simulink model "Full_stack_ADMM"  (R2022b)
settings: Solver=VariableStepAuto  StartTime=0.0  StopTime=inf  RelTol=1e-3
libraries: modbusMatLib x12
settings Model: Creator=pppc  LastModifiedBy=pppc
settings SolverCC: AlgebraicLoopSolver=TrustRegion
settings DebuggingCC: UnconnectedInputMsg=warning  UnconnectedOutputMsg=warning  UnconnectedLineMsg=warning  SFMachineParentedDataDiag=warning
settings ModelReferenceCC: EnableRefExpFcnMdlSchedulingChecks=on
settings RTWCC: DLArmComputeVersion=19.05

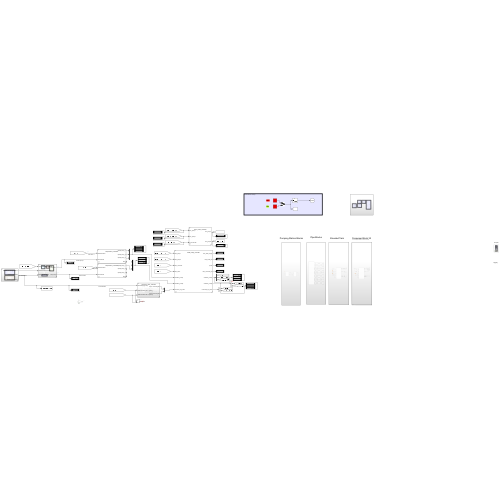
[thumbnail: Simulink's stored preview of the top-level diagram]
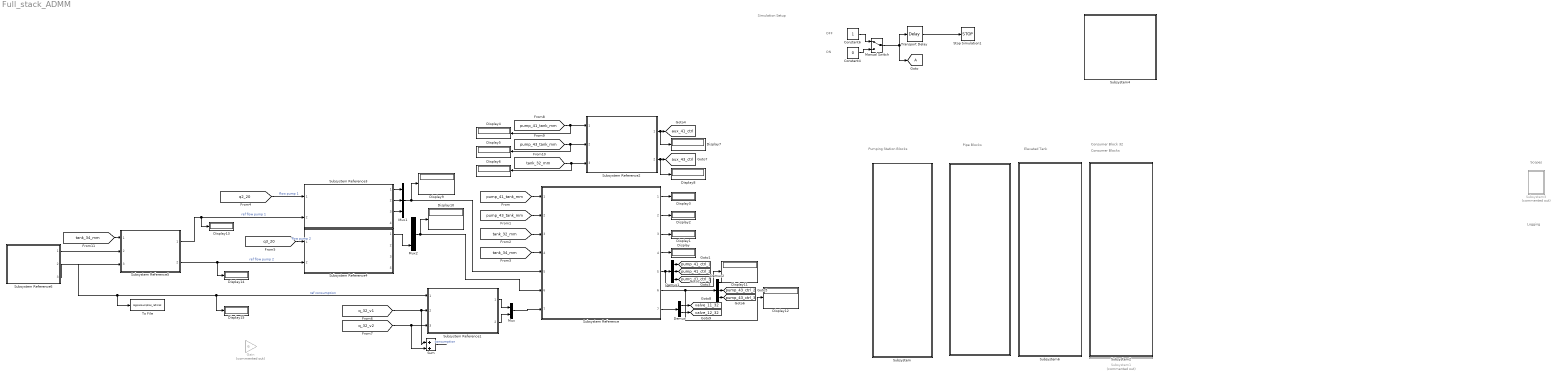
== system Full_stack_ADMM ==
  note: Logging
  note: Scopes
  note: Pumping Station Blocks
  note: OFF
  note: ON
  note: Simulation Setup
  note: Consumer Blocks
  note: Pipe Blocks
  note: Elevated Tank
  note: Consumer Block 32
  " " : Subsystem
  Constant4 : Constant  Value=0
  Constant6 : Constant
  Demux : Demux  Outputs=2
  Demux1 : Demux  Outputs=3
  Demux2 : Demux  Outputs=3
  Display{,1..15} (16 alike) : Display
  Gain : Gain  Commented=on  Gain=6
  Goto : Goto  TagVisibility=global
  Manual Switch : ManualSwitch
  Mux : Mux  Inputs=2
  Mux1 : Mux  Inputs=3
  Mux2 : Mux  Inputs=3
  Stop Simulation1 : Stop
  Subsystem : Subsystem
  Subsystem Reference : Subsystem  ReferencedSubsystem=WDN_safety_controller  consumer_tank_max=575  consumer_tank_min=75  pump_tank_min=125
  Subsystem Reference1 : Subsystem  ReferencedSubsystem=consumer_valve_controller
  Subsystem Reference2 : Subsystem  ReferencedSubsystem=reutrn_water_controller  tank_pump_max=530  consumer_min=75  consumer_max=570  switch_time=60  tank_pump_ref=400
  Subsystem Reference3 : Subsystem  ReferencedSubsystem=Pumpstation_Controller  Speedlimit_Upper=95  Speedlimit_Lower=65  TotalPumps=3  Kp=6.5  Ki=3.25
  Subsystem Reference4 : Subsystem  ReferencedSubsystem=Pumpstation_Controller  Speedlimit_Upper=95  Speedlimit_Lower=65  TotalPumps=1  Kp=16  Ki=2
  Subsystem Reference5 : Subsystem  ReferencedSubsystem=consensusADMM
  Subsystem Reference6 : Subsystem  ReferencedSubsystem=DemandEletricityPrice
  Subsystem1 : Subsystem  Commented=on
  Subsystem2 : Subsystem
  Subsystem3 : Subsystem  Commented=on
  Subsystem4 : Subsystem
  Subsystem6 : Subsystem
  Sum : Sum  Inputs=|++
  To File : ToFile  Filename=log\consumption_ref.mat  MatrixName=con_ref  SaveFormat=Timeseries
  Transport Delay : TransportDelay  DelayTime=2
  tag scope: aux_41_ctrl=global, aux_43_ctrl=global, pump_41_ctrl_1=global, pump_41_ctrl_2=global, pump_41_ctrl_3=global, pump_43_ctrl_2=global, pump_43_ctrl_3=global, valve_11_32=global, valve_12_32=global
  wires:
  Constant4/1 -> Manual Switch/2
  Transport Delay/1 -> Stop Simulation1/1
  Constant6/1 -> Manual Switch/1
  Manual Switch/1 -> Goto/1, Transport Delay/1
  Subsystem Reference1/1 -> Mux/1
  Subsystem Reference1/2 -> Mux/2
  Mux/1 -> Subsystem Reference/7
  Subsystem Reference/7 -> Demux/1
  Subsystem Reference3/2 -> Mux1/2
  Subsystem Reference3/1 -> Mux1/1
  Subsystem Reference3/3 -> Mux1/3
  Mux2/1 -> Display10/1, Subsystem Reference/6
  Mux1/1 -> Subsystem Reference/5, Display9/1
  Subsystem Reference5/2 -> Display14/1, Subsystem Reference4/2  "ref flow pump 2"
  Subsystem Reference5/1 -> Display13/1, Subsystem Reference3/2  "ref flow pump 1"
  Subsystem Reference6/1 -> Subsystem Reference5/2
  Subsystem Reference6/3 -> Subsystem Reference5/3
  [pump_41_tank_mm] -> Subsystem Reference/1
  [pump_43_tank_mm] -> Subsystem Reference/2
  [tank_32_mm] -> Subsystem Reference/3
  [tank_34_mm] -> Subsystem Reference/4
  [q2_20] -> Subsystem Reference3/1  "flow pump 1"
  [q3_20] -> Subsystem Reference4/1  "flow pump 2"
  [q_32_v1] -> Sum/1, Subsystem Reference1/2
  [q_32_v2] -> Sum/2, Subsystem Reference1/3
  [pump_41_tank_mm] -> Display4/1, Subsystem Reference2/1
  [pump_43_tank_mm] -> Display5/1, Subsystem Reference2/2
  [tank_32_mm] -> Display6/1, Subsystem Reference2/3
  Subsystem Reference/5 -> Display11/1, Demux1/1
  Demux1/1 -> [pump_41_ctrl_1]
  Demux1/2 -> [pump_41_ctrl_2]
  Demux1/3 -> [pump_41_ctrl_3]
  [tank_34_mm] -> Subsystem Reference5/1
  Demux2/3 -> [pump_43_ctrl_3]
  Subsystem Reference/6 -> Demux2/1, Display12/1
  Demux2/1 -> ?
  Demux2/2 -> [pump_43_ctrl_2]
  Subsystem Reference/4 -> Display/1
  Subsystem Reference/3 -> Display1/1
  Subsystem Reference/2 -> Display2/1
  Subsystem Reference/1 -> Display3/1
  Subsystem Reference2/1 -> Display7/1, [aux_41_ctrl]
  Subsystem Reference2/2 -> Display8/1, [aux_43_ctrl]
  Demux/1 -> [valve_11_32]
  Demux/2 -> [valve_12_32]
  Sum/1 -> ?  "consumption"
  Subsystem Reference6/2 -> Display15/1, Subsystem Reference1/1, To File/1  "ref consumption"
  Subsystem Reference4/1 -> Mux2/3

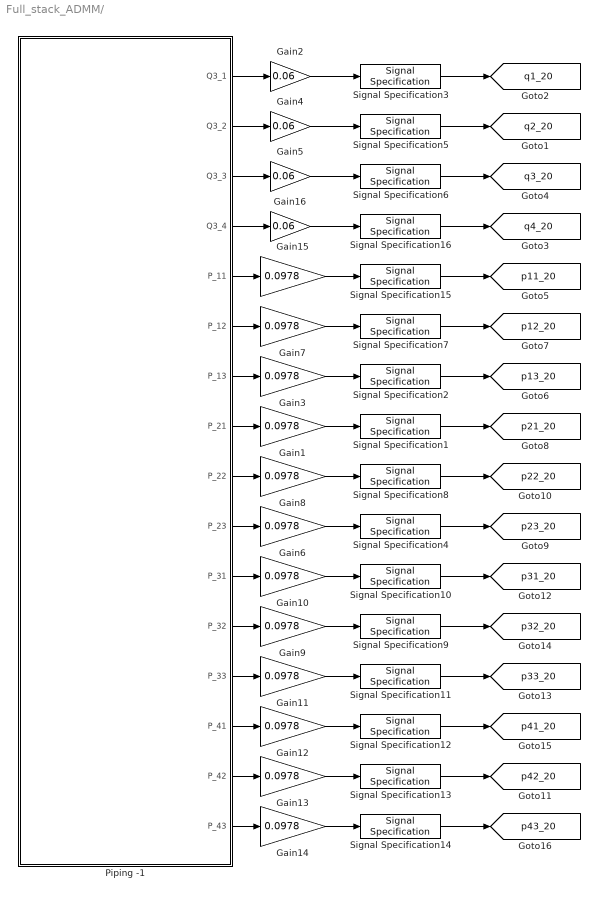
== system Full_stack_ADMM/  ==
  Gain{1,3,6..15} (12 alike) : Gain  Gain=0.0978
  Gain{2,4..5,16} (4 alike) : Gain  Gain=0.06
  Piping -1 : Subsystem
  Signal Specification{1..2,4,7..15} (12 alike) : SignalSpecification  Unit=bar
  Signal Specification{3,5..6,16} (4 alike) : SignalSpecification  Unit=m^3/hr
  tag scope: p11_20=global, p12_20=global, p13_20=global, p21_20=global, p22_20=global, p23_20=global, p31_20=global, p32_20=global, p33_20=global, p41_20=global, p42_20=global, p43_20=global, q1_20=global, q2_20=global, q3_20=global, q4_20=global
  wires:
  Gain8/1 -> Signal Specification8/1
  Piping -1/6(P_12) -> Gain7/1
  Gain5/1 -> Signal Specification6/1
  Gain9/1 -> Signal Specification9/1
  Piping -1/12(P_32) -> Gain9/1
  Piping -1/9(P_22) -> Gain8/1
  Piping -1/3(Q3_3) -> Gain5/1
  Piping -1/2(Q3_2) -> Gain4/1
  Gain7/1 -> Signal Specification7/1
  Gain4/1 -> Signal Specification5/1
  Gain16/1 -> Signal Specification16/1
  Piping -1/4(Q3_4) -> Gain16/1
  Piping -1/1(Q3_1) -> Gain2/1
  Piping -1/8(P_21) -> Gain1/1
  Gain1/1 -> Signal Specification1/1
  Gain2/1 -> Signal Specification3/1
  Gain3/1 -> Signal Specification2/1
  Piping -1/7(P_13) -> Gain3/1
  Piping -1/10(P_23) -> Gain6/1
  Gain6/1 -> Signal Specification4/1
  Gain10/1 -> Signal Specification10/1
  Piping -1/11(P_31) -> Gain10/1
  Gain11/1 -> Signal Specification11/1
  Gain12/1 -> Signal Specification12/1
  Piping -1/13(P_33) -> Gain11/1
  Piping -1/14(P_41) -> Gain12/1
  Gain13/1 -> Signal Specification13/1
  Piping -1/15(P_42) -> Gain13/1
  Gain14/1 -> Signal Specification14/1
  Piping -1/16(P_43) -> Gain14/1
  Gain15/1 -> Signal Specification15/1
  Piping -1/5(P_11) -> Gain15/1
  Signal Specification3/1 -> [q1_20]
  Signal Specification5/1 -> [q2_20]
  Signal Specification6/1 -> [q3_20]
  Signal Specification16/1 -> [q4_20]
  Signal Specification2/1 -> [p13_20]
  Signal Specification15/1 -> [p11_20]
  Signal Specification7/1 -> [p12_20]
  Signal Specification8/1 -> [p22_20]
  Signal Specification4/1 -> [p23_20]
  Signal Specification1/1 -> [p21_20]
  Signal Specification13/1 -> [p42_20]
  Signal Specification12/1 -> [p41_20]
  Signal Specification14/1 -> [p43_20]
  Signal Specification9/1 -> [p32_20]
  Signal Specification11/1 -> [p33_20]
  Signal Specification10/1 -> [p31_20]

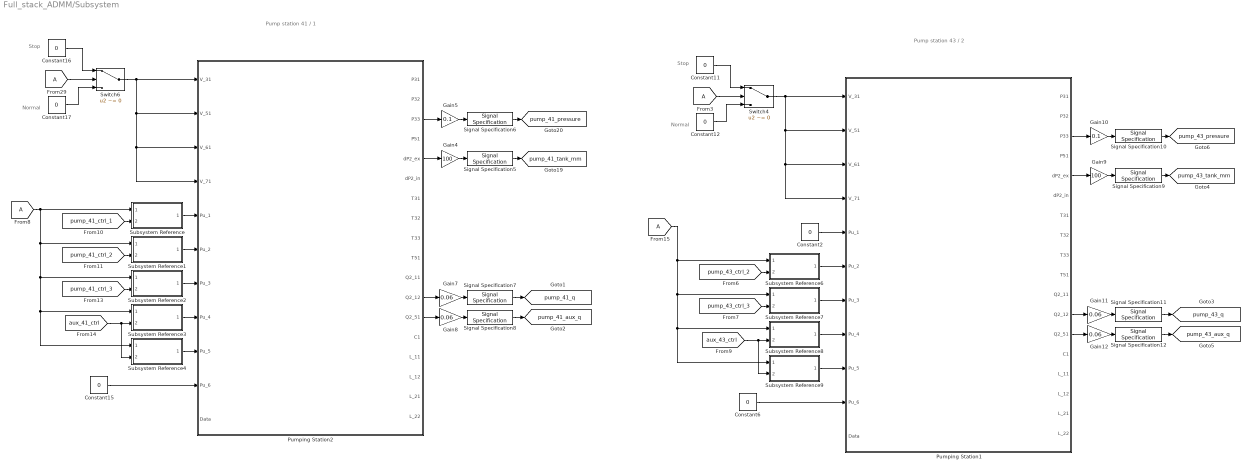
== system Full_stack_ADMM/Subsystem ==
  note: Stop
  note: Normal
  note: Pump station 41 / 1
  note: Normal
  note: Stop
  note: Pump station 43 / 2
  Constant{2,6,11..12,15..17} (7 alike) : Constant  Value=0
  From{3,8,15,29} (4 alike) : From  TagVisibility=global
  Gain10 : Gain  Gain=0.1
  Gain{7..8,11..12} (4 alike) : Gain  Gain=0.06
  Gain4 : Gain  Gain=100
  Gain5 : Gain  Gain=0.1
  Gain9 : Gain  Gain=100
  Pumping Station1 : Subsystem
  Pumping Station2 : Subsystem
  Signal Specification10 : SignalSpecification  Unit=bar
  Signal Specification{7..8,11..12} (4 alike) : SignalSpecification  Unit=m^3/hr
  Signal Specification5 : SignalSpecification  Unit=mm
  Signal Specification6 : SignalSpecification  Unit=bar
  Signal Specification9 : SignalSpecification  Unit=mm
  Subsystem Reference{,1..4,6..9} (9 alike) : Subsystem  ReferencedSubsystem=turn_off_system
  Switch4 : Switch  Criteria=u2 ~= 0  SaturateOnIntegerOverflow=off  InputSameDT=off
  Switch6 : Switch  Criteria=u2 ~= 0  SaturateOnIntegerOverflow=off  InputSameDT=off
  tag scope: pump_41_aux_q=global, pump_41_pressure=global, pump_41_q=global, pump_41_tank_mm=global, pump_43_aux_q=global, pump_43_pressure=global, pump_43_q=global, pump_43_tank_mm=global
  wires:
  Signal Specification6/1 -> [pump_41_pressure]
  Pumping Station2/5(dP2_ex) -> Gain4/1
  Switch6/1 -> Pumping Station2/4(V_71), Pumping Station2/3(V_61), Pumping Station2/2(V_51), Pumping Station2/1(V_31)
  Signal Specification5/1 -> [pump_41_tank_mm]
  From29/1 -> Switch6/2
  Constant17/1 -> Switch6/3
  Constant16/1 -> Switch6/1
  Gain5/1 -> Signal Specification6/1
  Gain4/1 -> Signal Specification5/1
  Pumping Station2/3(P33) -> Gain5/1
  Constant15/1 -> Pumping Station2/10(Pu_6)
  Gain8/1 -> Signal Specification8/1
  Signal Specification8/1 -> [pump_41_aux_q]
  Pumping Station2/13(Q2_51) -> Gain8/1
  Pumping Station2/12(Q2_12) -> Gain7/1
  Gain7/1 -> Signal Specification7/1
  Signal Specification7/1 -> [pump_41_q]
  Constant12/1 -> Switch4/3
  Signal Specification11/1 -> [pump_43_q]
  Switch4/1 -> Pumping Station1/4(V_71), Pumping Station1/3(V_61), Pumping Station1/2(V_51), Pumping Station1/1(V_31)
  Pumping Station1/12(Q2_12) -> Gain11/1
  Pumping Station1/13(Q2_51) -> Gain12/1
  Constant11/1 -> Switch4/1
  Gain10/1 -> Signal Specification10/1
  Pumping Station1/3(P33) -> Gain10/1
  Constant6/1 -> Pumping Station1/10(Pu_6)
  Gain11/1 -> Signal Specification11/1
  From3/1 -> Switch4/2
  Gain9/1 -> Signal Specification9/1
  Signal Specification12/1 -> [pump_43_aux_q]
  Signal Specification9/1 -> [pump_43_tank_mm]
  Signal Specification10/1 -> [pump_43_pressure]
  Gain12/1 -> Signal Specification12/1
  Pumping Station1/5(dP2_ex) -> Gain9/1
  Subsystem Reference/1 -> Pumping Station2/5(Pu_1)
  Subsystem Reference1/1 -> Pumping Station2/6(Pu_2)
  Subsystem Reference2/1 -> Pumping Station2/7(Pu_3)
  Subsystem Reference3/1 -> Pumping Station2/8(Pu_4)
  Subsystem Reference4/1 -> Pumping Station2/9(Pu_5)
  From8/1 -> Subsystem Reference4/1, Subsystem Reference3/1, Subsystem Reference2/1, Subsystem Reference1/1, Subsystem Reference/1
  [pump_41_ctrl_1] -> Subsystem Reference/2
  [pump_41_ctrl_2] -> Subsystem Reference1/2
  [pump_41_ctrl_3] -> Subsystem Reference2/2
  [aux_41_ctrl] -> Subsystem Reference4/2, Subsystem Reference3/2
  [aux_43_ctrl] -> Subsystem Reference9/2, Subsystem Reference8/2
  [pump_43_ctrl_3] -> Subsystem Reference7/2
  [pump_43_ctrl_2] -> Subsystem Reference6/2
  From15/1 -> Subsystem Reference9/1, Subsystem Reference8/1, Subsystem Reference7/1, Subsystem Reference6/1
  Subsystem Reference6/1 -> Pumping Station1/6(Pu_2)
  Subsystem Reference7/1 -> Pumping Station1/7(Pu_3)
  Subsystem Reference8/1 -> Pumping Station1/8(Pu_4)
  Subsystem Reference9/1 -> Pumping Station1/9(Pu_5)
  Constant2/1 -> Pumping Station1/5(Pu_1)

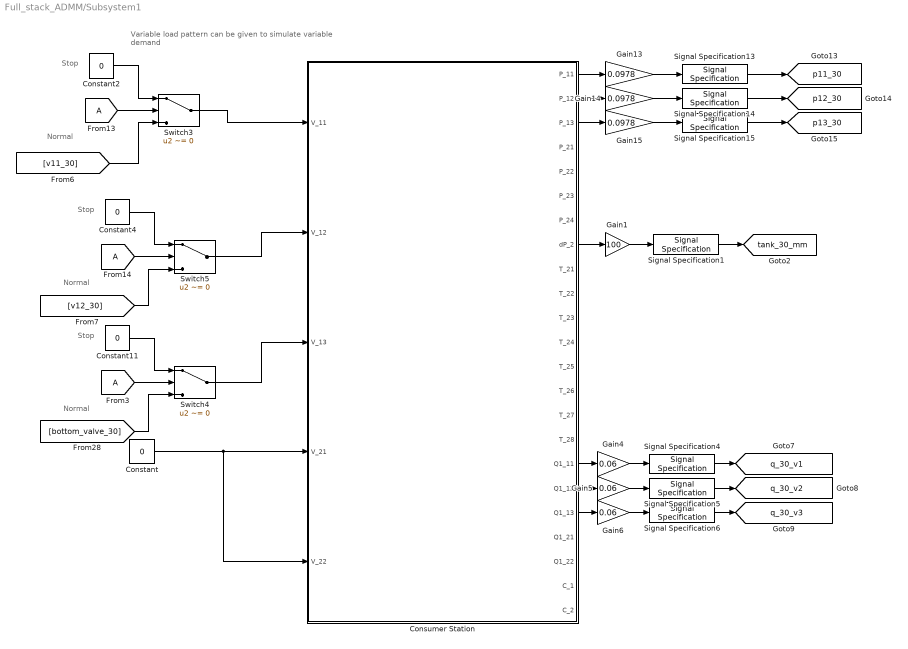
== system Full_stack_ADMM/Subsystem1 ==
  note: Variable load pattern can be
      | given to simulate variable demand
  note: Normal
  note: Normal
  note: Stop
  note: Stop
  note: Stop
  note: Normal
  Constant{,2,4,11} (4 alike) : Constant  Value=0
  Consumer Station : Subsystem
  From13 : From  TagVisibility=global
  From14 : From  TagVisibility=global
  From3 : From  TagVisibility=global
  Gain1 : Gain  Gain=100
  Gain13 : Gain  Gain=0.0978
  Gain14 : Gain  Gain=0.0978
  Gain15 : Gain  Gain=0.0978
  Gain4 : Gain  Gain=0.06
  Gain5 : Gain  Gain=0.06
  Gain6 : Gain  Gain=0.06
  Signal Specification1 : SignalSpecification  Unit=mm
  Signal Specification13 : SignalSpecification  Unit=bar
  Signal Specification14 : SignalSpecification  Unit=bar
  Signal Specification15 : SignalSpecification  Unit=bar
  Signal Specification4 : SignalSpecification  Unit=m^3/hr
  Signal Specification5 : SignalSpecification  Unit=m^3/hr
  Signal Specification6 : SignalSpecification  Unit=m^3/hr
  Switch3 : Switch  Criteria=u2 ~= 0  SaturateOnIntegerOverflow=off  InputSameDT=off
  Switch4 : Switch  Criteria=u2 ~= 0  SaturateOnIntegerOverflow=off  InputSameDT=off
  Switch5 : Switch  Criteria=u2 ~= 0  SaturateOnIntegerOverflow=off  InputSameDT=off
  tag scope: p11_30=global, p12_30=global, p13_30=global, q_30_v1=global, q_30_v2=global, q_30_v3=global, tank_30_mm=global
  wires:
  Gain14/1 -> Signal Specification14/1
  Signal Specification15/1 -> [p13_30]
  Signal Specification14/1 -> [p12_30]
  Signal Specification13/1 -> [p11_30]
  Gain13/1 -> Signal Specification13/1
  Consumer Station/2(P_12) -> Gain14/1
  Consumer Station/1(P_11) -> Gain13/1
  Signal Specification5/1 -> [q_30_v2]
  Gain5/1 -> Signal Specification5/1
  Gain4/1 -> Signal Specification4/1
  [bottom_valve_30] -> Switch4/3
  Constant11/1 -> Switch4/1
  Signal Specification4/1 -> [q_30_v1]
  Switch4/1 -> Consumer Station/3(V_13)
  Consumer Station/18(Q1_12) -> Gain5/1
  From13/1 -> Switch3/2
  Gain6/1 -> Signal Specification6/1
  Gain15/1 -> Signal Specification15/1
  Consumer Station/8(dP_2) -> Gain1/1
  Consumer Station/17(Q1_11) -> Gain4/1
  Switch3/1 -> Consumer Station/1(V_11)
  Signal Specification6/1 -> [q_30_v3]
  [v11_30] -> Switch3/3
  Signal Specification1/1 -> [tank_30_mm]
  Switch5/1 -> Consumer Station/2(V_12)
  [v12_30] -> Switch5/3
  Gain1/1 -> Signal Specification1/1
  From3/1 -> Switch4/2
  Constant/1 -> Consumer Station/5(V_22), Consumer Station/4(V_21)
  Constant4/1 -> Switch5/1
  Consumer Station/3(P_13) -> Gain15/1
  Consumer Station/19(Q1_13) -> Gain6/1
  Constant2/1 -> Switch3/1
  From14/1 -> Switch5/2

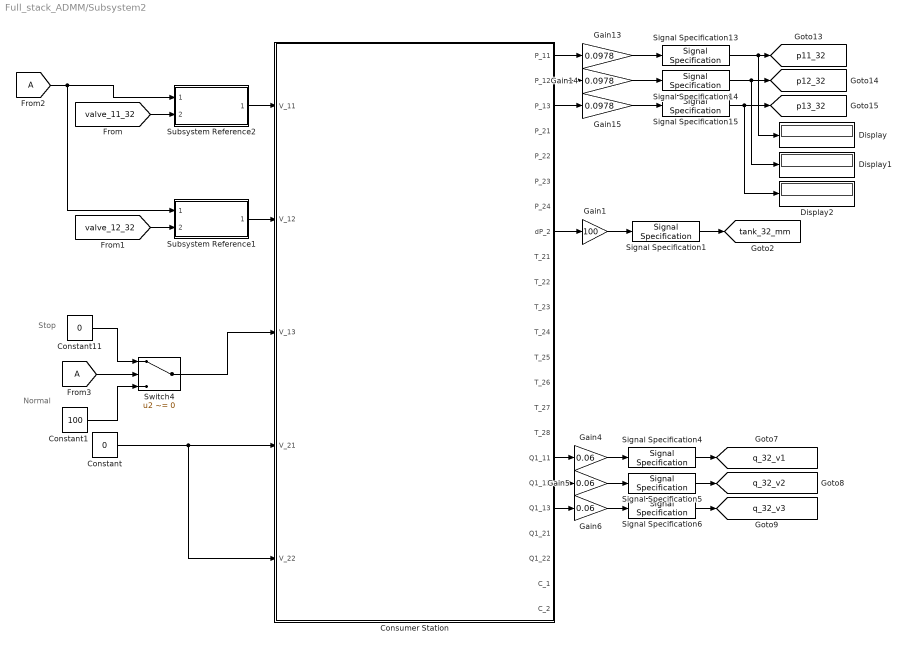
== system Full_stack_ADMM/Subsystem2 ==
  note: Stop
  note: Normal
  Constant : Constant  Value=0
  Constant1 : Constant  Value=100
  Constant11 : Constant  Value=0
  Consumer Station : Subsystem
  Display : Display
  Display1 : Display
  Display2 : Display
  From2 : From  TagVisibility=global
  From3 : From  TagVisibility=global
  Gain1 : Gain  Gain=100
  Gain13 : Gain  Gain=0.0978
  Gain14 : Gain  Gain=0.0978
  Gain15 : Gain  Gain=0.0978
  Gain4 : Gain  Gain=0.06
  Gain5 : Gain  Gain=0.06
  Gain6 : Gain  Gain=0.06
  Signal Specification1 : SignalSpecification  Unit=mm
  Signal Specification13 : SignalSpecification  Unit=bar
  Signal Specification14 : SignalSpecification  Unit=bar
  Signal Specification15 : SignalSpecification  Unit=bar
  Signal Specification4 : SignalSpecification  Unit=m^3/hr
  Signal Specification5 : SignalSpecification  Unit=m^3/hr
  Signal Specification6 : SignalSpecification  Unit=m^3/hr
  Subsystem Reference1 : Subsystem  ReferencedSubsystem=turn_off_system
  Subsystem Reference2 : Subsystem  ReferencedSubsystem=turn_off_system
  Switch4 : Switch  Criteria=u2 ~= 0  SaturateOnIntegerOverflow=off  InputSameDT=off
  tag scope: p11_32=global, p12_32=global, p13_32=global, q_32_v1=global, q_32_v2=global, q_32_v3=global, tank_32_mm=global
  wires:
  Consumer Station/19(Q1_13) -> Gain6/1
  Consumer Station/3(P_13) -> Gain15/1
  Constant/1 -> Consumer Station/4(V_21), Consumer Station/5(V_22)
  From3/1 -> Switch4/2
  Gain1/1 -> Signal Specification1/1
  Signal Specification1/1 -> [tank_32_mm]
  Signal Specification6/1 -> [q_32_v3]
  Consumer Station/17(Q1_11) -> Gain4/1
  Consumer Station/8(dP_2) -> Gain1/1
  Gain15/1 -> Signal Specification15/1
  Gain6/1 -> Signal Specification6/1
  Consumer Station/18(Q1_12) -> Gain5/1
  Switch4/1 -> Consumer Station/3(V_13)
  Signal Specification4/1 -> [q_32_v1]
  Constant11/1 -> Switch4/1
  Gain4/1 -> Signal Specification4/1
  Gain5/1 -> Signal Specification5/1
  Signal Specification5/1 -> [q_32_v2]
  Consumer Station/1(P_11) -> Gain13/1
  Consumer Station/2(P_12) -> Gain14/1
  Gain13/1 -> Signal Specification13/1
  Signal Specification13/1 -> Display/1, [p11_32]
  Signal Specification14/1 -> Display1/1, [p12_32]
  Signal Specification15/1 -> Display2/1, [p13_32]
  Gain14/1 -> Signal Specification14/1
  Constant1/1 -> Switch4/3
  Subsystem Reference1/1 -> Consumer Station/2(V_12)
  Subsystem Reference2/1 -> Consumer Station/1(V_11)
  [valve_11_32] -> Subsystem Reference2/2
  [valve_12_32] -> Subsystem Reference1/2
  From2/1 -> Subsystem Reference1/1, Subsystem Reference2/1

== system Full_stack_ADMM/Subsystem3 ==
  note: TO WORKSPACE
  note: Pumping scopes
  note: Demand scopes
  note: Reservoir scopes
  Consumer tank : Scope  Commented=on  NumInputPorts=3
  Elevated reservoir : Scope  Commented=on  NumInputPorts=2
  Flow of auxillary pump : Scope  Commented=on  NumInputPorts=2
  From10 : From  Commented=on  GotoTag=resvr_tank_mm
  From11 : From  Commented=on  GotoTag=resvr_tank_q
  From13 : From  Commented=on  GotoTag=pump_1_ctrl  TagVisibility=global
  From15 : From  Commented=on  GotoTag=d1_q
  From16 : From  Commented=on  GotoTag=d2_q
  From17 : From  Commented=on  GotoTag=dem_tank_out_q
  From18 : From  Commented=on  GotoTag=pump_1_q  TagVisibility=global
  From19 : From  Commented=on  GotoTag=pump_aux_q  TagVisibility=global
  From20 : From  Commented=on  GotoTag=pump_1_q_mag
  From22 : From  Commented=on  GotoTag=pump_tank_mm  TagVisibility=global
  From23 : From  Commented=on  GotoTag=pipe_3_q_mag
  From24 : From  Commented=on  GotoTag=supply_pressure  TagVisibility=global
  From25 : From  Commented=on  GotoTag=pump_1_q_mag
  From26 : From  Commented=on  GotoTag=pump_1_ctrl  TagVisibility=global
  From6 : From  Commented=on  GotoTag=aux_ctrl
  From8 : From  Commented=on  GotoTag=dem_tank_mm
  Level of pump external tank : Scope  Commented=on  NumInputPorts=4
  Mux1 : Mux  Commented=on  Inputs=2
  Mux2 : Mux  Commented=on  Inputs=2
  Pipe flow : Scope  Commented=on
  To Workspace : ToWorkspace  Commented=on  VariableName=pump_control  SampleTime=-1
      settings: Save2DSignal=2-D array (concatenate along first dimension)
  To Workspace1 : ToWorkspace  Commented=on  VariableName=flow  SampleTime=-1
      settings: Save2DSignal=2-D array (concatenate along first dimension)
  wires:
  From15/1 -> Mux1/1
  From22/1 -> Level of pump external tank/1
  From11/1 -> Elevated reservoir/2
  From8/1 -> Consumer tank/1
  Mux1/1 -> Consumer tank/3
  From16/1 -> Mux1/2
  From18/1 -> Mux2/1
  From24/1 -> Level of pump external tank/2
  From20/1 -> Mux2/2
  From23/1 -> Pipe flow/1
  From26/1 -> To Workspace/1
  From10/1 -> Elevated reservoir/1
  From13/1 -> Level of pump external tank/4
  From19/1 -> Flow of auxillary pump/1
  From17/1 -> Consumer tank/2
  From6/1 -> Flow of auxillary pump/2
  Mux2/1 -> Level of pump external tank/3
  From25/1 -> To Workspace1/1

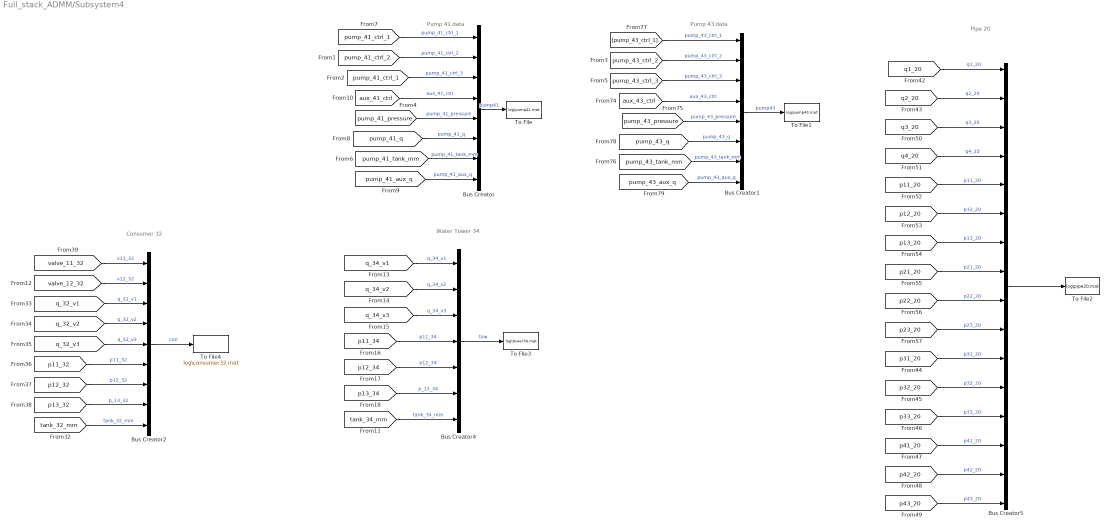
== system Full_stack_ADMM/Subsystem4 ==
  note: Pipe 20
  note: Pump 41 data
  note: Consumer 32
  note: Pump 43 data
  note: Water Tower 34
  Bus Creator : BusCreator  Inputs=8
  Bus Creator1 : BusCreator  Inputs=8
  Bus Creator2 : BusCreator  Inputs=9
  Bus Creator4 : BusCreator  Inputs=7
  Bus Creator5 : BusCreator  Inputs=16
  To File : ToFile  Filename=log\pump41.mat  MatrixName=pump41  SaveFormat=Timeseries
  To File1 : ToFile  Filename=log\pump43.mat  MatrixName=pump43  SaveFormat=Timeseries
  To File2 : ToFile  Filename=log\pipe20.mat  MatrixName=pipe20  SaveFormat=Timeseries
  To File3 : ToFile  Filename=log\tower34.mat  MatrixName=tow34  SaveFormat=Timeseries
  To File4 : ToFile  Filename=log\consumer32.mat  MatrixName=con32  SaveFormat=Timeseries
  wires:
  [pump_41_tank_mm] -> Bus Creator/7  "pump_41_tank_mm"
  [aux_41_ctrl] -> Bus Creator/4  "aux_41_ctrl"
  [pump_41_aux_q] -> Bus Creator/8  "pump_41_aux_q"
  [pump_41_pressure] -> Bus Creator/5  "pump_41_pressure"
  [pump_41_ctrl_1] -> Bus Creator/1  "pump_41_ctrl_1"
  [pump_41_q] -> Bus Creator/6  "pump_41_q"
  Bus Creator/1 -> To File/1  "pump41"
  [tank_32_mm] -> Bus Creator2/9  "tank_32_mm"
  [p13_32] -> Bus Creator2/8  "p_13_32"
  [q_32_v2] -> Bus Creator2/4  "q_32_v2"
  Bus Creator2/1 -> To File4/1  "con"
  [q_32_v1] -> Bus Creator2/3  "q_32_v1"
  [valve_11_32] -> Bus Creator2/1  "v11_32"
  [q_32_v3] -> Bus Creator2/5  "q_32_v3"
  [p11_32] -> Bus Creator2/6  "p11_32"
  [p12_32] -> Bus Creator2/7  "p12_32"
  [p43_20] -> Bus Creator5/16  "p43_20"
  [q1_20] -> Bus Creator5/1  "q1_20"
  [p42_20] -> Bus Creator5/15  "p42_20"
  [p41_20] -> Bus Creator5/14  "p41_20"
  [p33_20] -> Bus Creator5/13  "p33_20"
  [p32_20] -> Bus Creator5/12  "p32_20"
  [p31_20] -> Bus Creator5/11  "p31_20"
  [p23_20] -> Bus Creator5/10  "p23_20"
  [p22_20] -> Bus Creator5/9  "p22_20"
  [p21_20] -> Bus Creator5/8  "p21_20"
  [p13_20] -> Bus Creator5/7  "p13_20"
  [p12_20] -> Bus Creator5/6  "p12_20"
  [p11_20] -> Bus Creator5/5  "p11_20"
  [q4_20] -> Bus Creator5/4  "q4_20"
  [q3_20] -> Bus Creator5/3  "q3_20"
  [q2_20] -> Bus Creator5/2  "q2_20"
  Bus Creator5/1 -> To File2/1
  [pump_43_q] -> Bus Creator1/6  "pump_43_q"
  [aux_43_ctrl] -> Bus Creator1/4  "aux_43_ctrl"
  Bus Creator1/1 -> To File1/1  "pump43"
  [pump_43_ctrl_1] -> Bus Creator1/1  "pump_43_ctrl_1"
  [pump_43_tank_mm] -> Bus Creator1/7  "pump_43_tank_mm"
  [pump_43_aux_q] -> Bus Creator1/8  "pump_43_aux_q"
  [pump_43_pressure] -> Bus Creator1/5  "pump_43_pressure"
  [q_34_v2] -> Bus Creator4/2  "q_34_v2"
  [tank_34_mm] -> Bus Creator4/7  "tank_34_mm"
  [q_34_v3] -> Bus Creator4/3  "q_34_v3"
  [p11_34] -> Bus Creator4/4  "p11_34"
  Bus Creator4/1 -> To File3/1  "tow"
  [p13_34] -> Bus Creator4/6  "p_13_34"
  [p12_34] -> Bus Creator4/5  "p12_34"
  [q_34_v1] -> Bus Creator4/1  "q_34_v1"
  [pump_41_ctrl_2] -> Bus Creator/2  "pump_41_ctrl_2"
  [pump_41_ctrl_1] -> Bus Creator/3  "pump_41_ctrl_3"
  [pump_43_ctrl_2] -> Bus Creator1/2  "pump_43_ctrl_2"
  [pump_43_ctrl_3] -> Bus Creator1/3  "pump_43_ctrl_3"
  [valve_12_32] -> Bus Creator2/2  "v12_32"

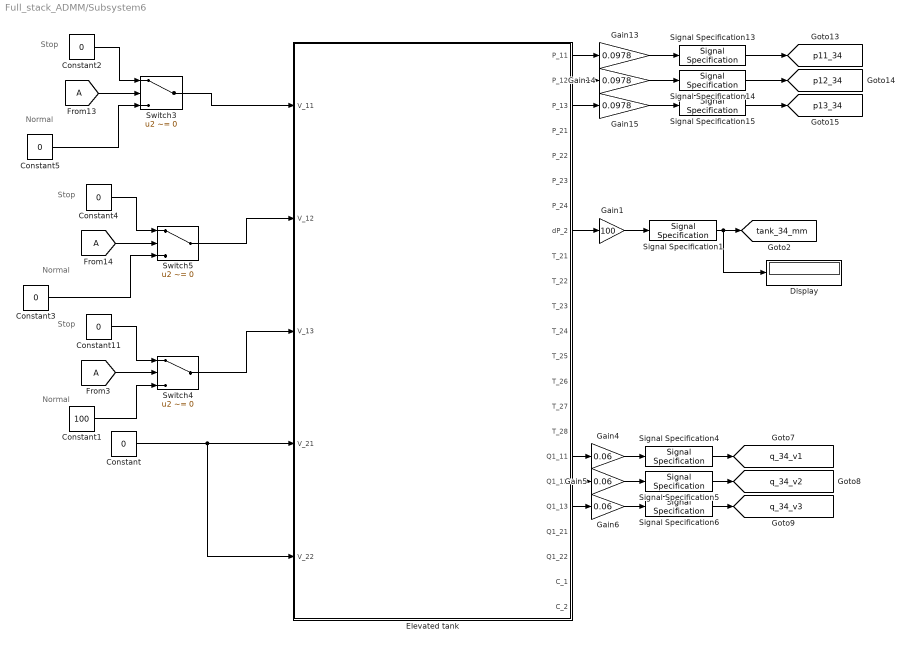
== system Full_stack_ADMM/Subsystem6 ==
  note: Normal
  note: Normal
  note: Stop
  note: Stop
  note: Stop
  note: Normal
  Constant{,2..5,11} (6 alike) : Constant  Value=0
  Constant1 : Constant  Value=100
  Display : Display
  Elevated tank : Subsystem
  From13 : From  TagVisibility=global
  From14 : From  TagVisibility=global
  From3 : From  TagVisibility=global
  Gain1 : Gain  Gain=100
  Gain13 : Gain  Gain=0.0978
  Gain14 : Gain  Gain=0.0978
  Gain15 : Gain  Gain=0.0978
  Gain4 : Gain  Gain=0.06
  Gain5 : Gain  Gain=0.06
  Gain6 : Gain  Gain=0.06
  Signal Specification1 : SignalSpecification  Unit=mm
  Signal Specification13 : SignalSpecification  Unit=bar
  Signal Specification14 : SignalSpecification  Unit=bar
  Signal Specification15 : SignalSpecification  Unit=bar
  Signal Specification4 : SignalSpecification  Unit=m^3/hr
  Signal Specification5 : SignalSpecification  Unit=m^3/hr
  Signal Specification6 : SignalSpecification  Unit=m^3/hr
  Switch3 : Switch  Criteria=u2 ~= 0  SaturateOnIntegerOverflow=off  InputSameDT=off
  Switch4 : Switch  Criteria=u2 ~= 0  SaturateOnIntegerOverflow=off  InputSameDT=off
  Switch5 : Switch  Criteria=u2 ~= 0  SaturateOnIntegerOverflow=off  InputSameDT=off
  tag scope: p11_34=global, p12_34=global, p13_34=global, q_34_v1=global, q_34_v2=global, q_34_v3=global, tank_34_mm=global
  wires:
  Gain14/1 -> Signal Specification14/1
  Signal Specification15/1 -> [p13_34]
  Signal Specification14/1 -> [p12_34]
  Signal Specification13/1 -> [p11_34]
  Gain13/1 -> Signal Specification13/1
  Elevated tank/2(P_12) -> Gain14/1
  Elevated tank/1(P_11) -> Gain13/1
  Signal Specification5/1 -> [q_34_v2]
  Gain5/1 -> Signal Specification5/1
  Gain4/1 -> Signal Specification4/1
  Constant11/1 -> Switch4/1
  Signal Specification4/1 -> [q_34_v1]
  Switch4/1 -> Elevated tank/3(V_13)
  Elevated tank/18(Q1_12) -> Gain5/1
  From13/1 -> Switch3/2
  Gain6/1 -> Signal Specification6/1
  Gain15/1 -> Signal Specification15/1
  Elevated tank/8(dP_2) -> Gain1/1
  Elevated tank/17(Q1_11) -> Gain4/1
  Switch3/1 -> Elevated tank/1(V_11)
  Signal Specification6/1 -> [q_34_v3]
  Constant5/1 -> Switch3/3
  Signal Specification1/1 -> Display/1, [tank_34_mm]
  Switch5/1 -> Elevated tank/2(V_12)
  Constant3/1 -> Switch5/3
  Gain1/1 -> Signal Specification1/1
  From3/1 -> Switch4/2
  Constant/1 -> Elevated tank/5(V_22), Elevated tank/4(V_21)
  Constant4/1 -> Switch5/1
  Elevated tank/3(P_13) -> Gain15/1
  Elevated tank/19(Q1_13) -> Gain6/1
  Constant2/1 -> Switch3/1
  From14/1 -> Switch5/2
  Constant1/1 -> Switch4/3

== system Full_stack_ADMM/ /Piping -1 ==
  note: Free
  Constant : Constant  Value=zeros(19,1)
  Demux : Demux  Outputs=[4 12 8]
  Demux1 : Demux
  Demux2 : Demux  Outputs=12
  Demux3 : Demux
  Modbus Read : modbusMatLib/Modbus Read  registry=0  ipAddress='192.168.100.20'  port=502
  Modbus Write : modbusMatLib/Modbus Write  registry=001  port=502  ipAddress='192.168.100.20'
  Q3_1 : Outport  VectorParamsAs1DForOutWhenUnconnected=off
  Q3_2 : Outport  Port=2  VectorParamsAs1DForOutWhenUnconnected=off
  Q3_3 : Outport  Port=3  VectorParamsAs1DForOutWhenUnconnected=off
  Q3_4 : Outport  Port=4  VectorParamsAs1DForOutWhenUnconnected=off
  P_11 : Outport  Port=5  VectorParamsAs1DForOutWhenUnconnected=off
  P_12 : Outport  Port=6  VectorParamsAs1DForOutWhenUnconnected=off
  P_13 : Outport  Port=7  VectorParamsAs1DForOutWhenUnconnected=off
  P_21 : Outport  Port=8  VectorParamsAs1DForOutWhenUnconnected=off
  P_22 : Outport  Port=9  VectorParamsAs1DForOutWhenUnconnected=off
  P_23 : Outport  Port=10  VectorParamsAs1DForOutWhenUnconnected=off
  P_31 : Outport  Port=11  VectorParamsAs1DForOutWhenUnconnected=off
  P_32 : Outport  Port=12  VectorParamsAs1DForOutWhenUnconnected=off
  P_33 : Outport  Port=13  VectorParamsAs1DForOutWhenUnconnected=off
  P_41 : Outport  Port=14  VectorParamsAs1DForOutWhenUnconnected=off
  P_42 : Outport  Port=15  VectorParamsAs1DForOutWhenUnconnected=off
  P_43 : Outport  Port=16  VectorParamsAs1DForOutWhenUnconnected=off
  wires:
  Demux1/4 -> Q3_4/1
  Demux1/2 -> Q3_2/1
  Demux1/1 -> Q3_1/1
  Demux1/3 -> Q3_3/1
  Demux/1 -> Demux1/1
  Modbus Read/1 -> Demux/1
  Constant/1 -> Modbus Write/1
  Demux/2 -> Demux2/1
  Demux/3 -> Demux3/1
  Demux2/1 -> P_11/1
  Demux2/2 -> P_12/1
  Demux2/3 -> P_13/1
  Demux2/4 -> P_21/1
  Demux2/5 -> P_22/1
  Demux2/6 -> P_23/1
  Demux2/7 -> P_31/1
  Demux2/8 -> P_32/1
  Demux2/9 -> P_33/1
  Demux2/10 -> P_41/1
  Demux2/11 -> P_42/1
  Demux2/12 -> P_43/1

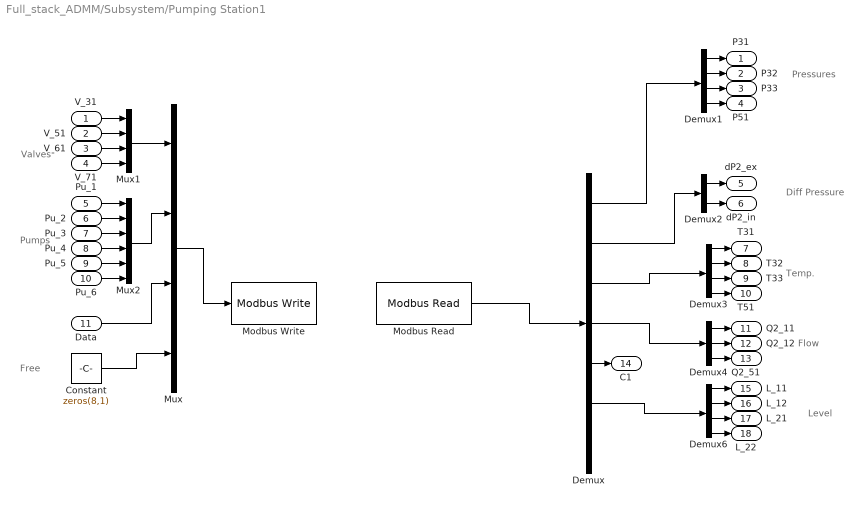
== system Full_stack_ADMM/Subsystem/Pumping Station1 ==
  note: Free
  note: Pumps
  note: Valves
  note: Flow
  note: Temp.
  note: Diff Pressure
  note: Pressures
  note: Level
  V_31 : Inport
  V_51 : Inport  Port=2
  V_61 : Inport  Port=3
  V_71 : Inport  Port=4
  Pu_1 : Inport  Port=5
  Pu_2 : Inport  Port=6
  Pu_3 : Inport  Port=7
  Pu_4 : Inport  Port=8
  Pu_5 : Inport  Port=9
  Pu_6 : Inport  Port=10
  Data : Inport  Port=11
  Constant : Constant  Value=zeros(8,1)
  Demux : Demux  Outputs=[4 2 4 3 1 4 6]
  Demux1 : Demux
  Demux2 : Demux  Outputs=2
  Demux3 : Demux
  Demux4 : Demux  Outputs=3
  Demux6 : Demux
  Modbus Read : modbusMatLib/Modbus Read  registry=0  ipAddress='192.168.100.43'  port=502
  Modbus Write : modbusMatLib/Modbus Write  registry=001  port=502  ipAddress='192.168.100.43'
  Mux : Mux
  Mux1 : Mux
  Mux2 : Mux  Inputs=6
  P31 : Outport  VectorParamsAs1DForOutWhenUnconnected=off
  P32 : Outport  Port=2  VectorParamsAs1DForOutWhenUnconnected=off
  P33 : Outport  Port=3  VectorParamsAs1DForOutWhenUnconnected=off
  P51 : Outport  Port=4  VectorParamsAs1DForOutWhenUnconnected=off
  dP2_ex : Outport  Port=5  VectorParamsAs1DForOutWhenUnconnected=off
  dP2_in : Outport  Port=6  VectorParamsAs1DForOutWhenUnconnected=off
  T31 : Outport  Port=7  VectorParamsAs1DForOutWhenUnconnected=off
  T32 : Outport  Port=8  VectorParamsAs1DForOutWhenUnconnected=off
  T33 : Outport  Port=9  VectorParamsAs1DForOutWhenUnconnected=off
  T51 : Outport  Port=10  VectorParamsAs1DForOutWhenUnconnected=off
  Q2_11 : Outport  Port=11  VectorParamsAs1DForOutWhenUnconnected=off
  Q2_12 : Outport  Port=12  VectorParamsAs1DForOutWhenUnconnected=off
  Q2_51 : Outport  Port=13  VectorParamsAs1DForOutWhenUnconnected=off
  C1 : Outport  Port=14  VectorParamsAs1DForOutWhenUnconnected=off
  L_11 : Outport  Port=15  VectorParamsAs1DForOutWhenUnconnected=off
  L_12 : Outport  Port=16  VectorParamsAs1DForOutWhenUnconnected=off
  L_21 : Outport  Port=17  VectorParamsAs1DForOutWhenUnconnected=off
  L_22 : Outport  Port=18  VectorParamsAs1DForOutWhenUnconnected=off
  wires:
  Demux4/1 -> Q2_11/1
  Demux/2 -> Demux2/1
  Demux/4 -> Demux4/1
  Demux2/1 -> dP2_ex/1
  Demux/3 -> Demux3/1
  Demux/6 -> Demux6/1
  Demux/1 -> Demux1/1
  Demux3/4 -> T51/1
  Demux1/4 -> P51/1
  Demux3/2 -> T32/1
  Modbus Read/1 -> Demux/1
  Demux6/1 -> L_11/1
  Demux6/2 -> L_12/1
  Demux4/3 -> Q2_51/1
  Demux4/2 -> Q2_12/1
  Demux6/3 -> L_21/1
  Demux6/4 -> L_22/1
  Demux3/3 -> T33/1
  Demux1/1 -> P31/1
  Demux1/2 -> P32/1
  Demux/5 -> C1/1
  Demux1/3 -> P33/1
  Demux2/2 -> dP2_in/1
  Demux3/1 -> T31/1
  Mux/1 -> Modbus Write/1
  Mux1/1 -> Mux/1
  V_31/1 -> Mux1/1
  V_51/1 -> Mux1/2
  V_61/1 -> Mux1/3
  V_71/1 -> Mux1/4
  Pu_4/1 -> Mux2/4
  Pu_3/1 -> Mux2/3
  Pu_1/1 -> Mux2/1
  Pu_2/1 -> Mux2/2
  Mux2/1 -> Mux/2
  Pu_5/1 -> Mux2/5
  Pu_6/1 -> Mux2/6
  Data/1 -> Mux/3
  Constant/1 -> Mux/4

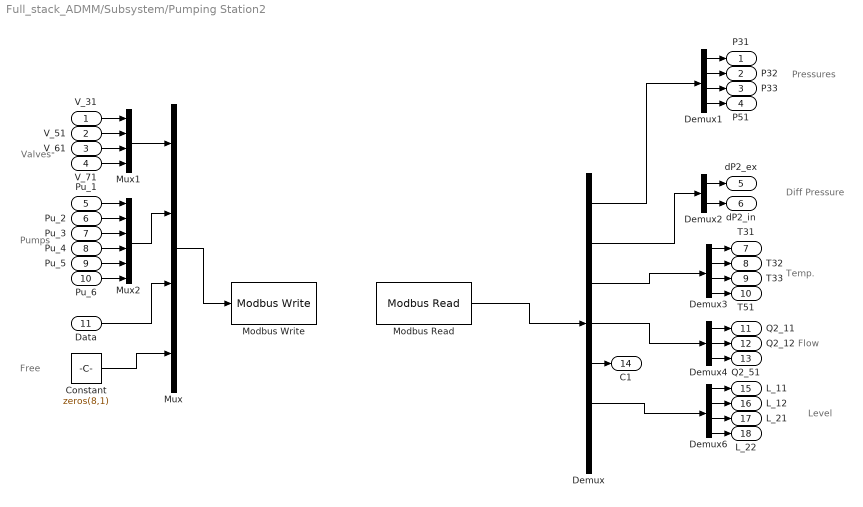
== system Full_stack_ADMM/Subsystem/Pumping Station2 ==
  note: Free
  note: Pumps
  note: Valves
  note: Flow
  note: Temp.
  note: Diff Pressure
  note: Pressures
  note: Level
  V_31 : Inport
  V_51 : Inport  Port=2
  V_61 : Inport  Port=3
  V_71 : Inport  Port=4
  Pu_1 : Inport  Port=5
  Pu_2 : Inport  Port=6
  Pu_3 : Inport  Port=7
  Pu_4 : Inport  Port=8
  Pu_5 : Inport  Port=9
  Pu_6 : Inport  Port=10
  Data : Inport  Port=11
  Constant : Constant  Value=zeros(8,1)
  Demux : Demux  Outputs=[4 2 4 3 1 4 6]
  Demux1 : Demux
  Demux2 : Demux  Outputs=2
  Demux3 : Demux
  Demux4 : Demux  Outputs=3
  Demux6 : Demux
  Modbus Read : modbusMatLib/Modbus Read  registry=0  ipAddress='192.168.100.41'  port=502
  Modbus Write : modbusMatLib/Modbus Write  registry=001  port=502  ipAddress='192.168.100.41'
  Mux : Mux
  Mux1 : Mux
  Mux2 : Mux  Inputs=6
  P31 : Outport  VectorParamsAs1DForOutWhenUnconnected=off
  P32 : Outport  Port=2  VectorParamsAs1DForOutWhenUnconnected=off
  P33 : Outport  Port=3  VectorParamsAs1DForOutWhenUnconnected=off
  P51 : Outport  Port=4  VectorParamsAs1DForOutWhenUnconnected=off
  dP2_ex : Outport  Port=5  VectorParamsAs1DForOutWhenUnconnected=off
  dP2_in : Outport  Port=6  VectorParamsAs1DForOutWhenUnconnected=off
  T31 : Outport  Port=7  VectorParamsAs1DForOutWhenUnconnected=off
  T32 : Outport  Port=8  VectorParamsAs1DForOutWhenUnconnected=off
  T33 : Outport  Port=9  VectorParamsAs1DForOutWhenUnconnected=off
  T51 : Outport  Port=10  VectorParamsAs1DForOutWhenUnconnected=off
  Q2_11 : Outport  Port=11  VectorParamsAs1DForOutWhenUnconnected=off
  Q2_12 : Outport  Port=12  VectorParamsAs1DForOutWhenUnconnected=off
  Q2_51 : Outport  Port=13  VectorParamsAs1DForOutWhenUnconnected=off
  C1 : Outport  Port=14  VectorParamsAs1DForOutWhenUnconnected=off
  L_11 : Outport  Port=15  VectorParamsAs1DForOutWhenUnconnected=off
  L_12 : Outport  Port=16  VectorParamsAs1DForOutWhenUnconnected=off
  L_21 : Outport  Port=17  VectorParamsAs1DForOutWhenUnconnected=off
  L_22 : Outport  Port=18  VectorParamsAs1DForOutWhenUnconnected=off
  wires:
  Demux4/1 -> Q2_11/1
  Demux/2 -> Demux2/1
  Demux/4 -> Demux4/1
  Demux2/1 -> dP2_ex/1
  Demux/3 -> Demux3/1
  Demux/6 -> Demux6/1
  Demux/1 -> Demux1/1
  Demux3/4 -> T51/1
  Demux1/4 -> P51/1
  Demux3/2 -> T32/1
  Modbus Read/1 -> Demux/1
  Demux6/1 -> L_11/1
  Demux6/2 -> L_12/1
  Demux4/3 -> Q2_51/1
  Demux4/2 -> Q2_12/1
  Demux6/3 -> L_21/1
  Demux6/4 -> L_22/1
  Demux3/3 -> T33/1
  Demux1/1 -> P31/1
  Demux1/2 -> P32/1
  Demux/5 -> C1/1
  Demux1/3 -> P33/1
  Demux2/2 -> dP2_in/1
  Demux3/1 -> T31/1
  Mux/1 -> Modbus Write/1
  Mux1/1 -> Mux/1
  V_31/1 -> Mux1/1
  V_51/1 -> Mux1/2
  V_61/1 -> Mux1/3
  V_71/1 -> Mux1/4
  Pu_4/1 -> Mux2/4
  Pu_3/1 -> Mux2/3
  Pu_1/1 -> Mux2/1
  Pu_2/1 -> Mux2/2
  Mux2/1 -> Mux/2
  Pu_5/1 -> Mux2/5
  Pu_6/1 -> Mux2/6
  Data/1 -> Mux/3
  Constant/1 -> Mux/4

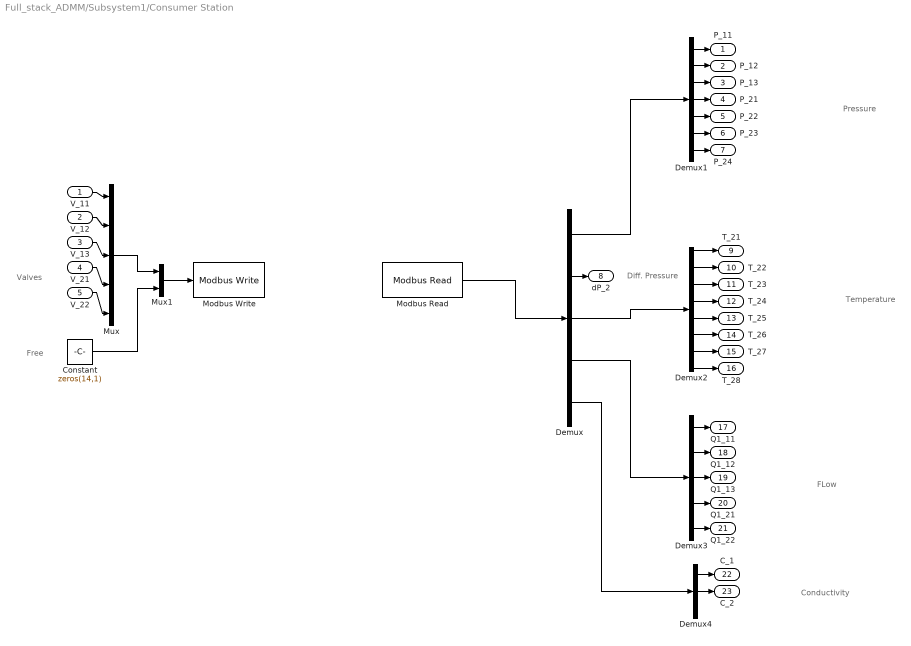
== system Full_stack_ADMM/Subsystem1/Consumer Station ==
  note: Pressure
  note: Temperature
  note: FLow
  note: Conductivity
  note: Valves
  note: Diff. Pressure
  note: Free
  V_11 : Inport
  V_12 : Inport  Port=2
  V_13 : Inport  Port=3
  V_21 : Inport  Port=4
  V_22 : Inport  Port=5
  Constant : Constant  Value=zeros(14,1)
  Demux : Demux  Outputs=[7 1 8 5 3]
  Demux1 : Demux  Outputs=7
  Demux2 : Demux  Outputs=8
  Demux3 : Demux  Outputs=5
  Demux4 : Demux  Outputs=3
  Modbus Read : modbusMatLib/Modbus Read  registry=0  ipAddress='192.168.100.30'  port=502
  Modbus Write : modbusMatLib/Modbus Write  registry=001  port=502  ipAddress='192.168.100.30'
  Mux : Mux  Inputs=5
  Mux1 : Mux  Inputs=2
  P_11 : Outport  VectorParamsAs1DForOutWhenUnconnected=off
  P_12 : Outport  Port=2  VectorParamsAs1DForOutWhenUnconnected=off
  P_13 : Outport  Port=3  VectorParamsAs1DForOutWhenUnconnected=off
  P_21 : Outport  Port=4  VectorParamsAs1DForOutWhenUnconnected=off
  P_22 : Outport  Port=5  VectorParamsAs1DForOutWhenUnconnected=off
  P_23 : Outport  Port=6  VectorParamsAs1DForOutWhenUnconnected=off
  P_24 : Outport  Port=7  VectorParamsAs1DForOutWhenUnconnected=off
  dP_2 : Outport  Port=8  VectorParamsAs1DForOutWhenUnconnected=off
  T_21 : Outport  Port=9  VectorParamsAs1DForOutWhenUnconnected=off
  T_22 : Outport  Port=10  VectorParamsAs1DForOutWhenUnconnected=off
  T_23 : Outport  Port=11  VectorParamsAs1DForOutWhenUnconnected=off
  T_24 : Outport  Port=12  VectorParamsAs1DForOutWhenUnconnected=off
  T_25 : Outport  Port=13  VectorParamsAs1DForOutWhenUnconnected=off
  T_26 : Outport  Port=14  VectorParamsAs1DForOutWhenUnconnected=off
  T_27 : Outport  Port=15  VectorParamsAs1DForOutWhenUnconnected=off
  T_28 : Outport  Port=16  VectorParamsAs1DForOutWhenUnconnected=off
  Q1_11 : Outport  Port=17  VectorParamsAs1DForOutWhenUnconnected=off
  Q1_12 : Outport  Port=18  VectorParamsAs1DForOutWhenUnconnected=off
  Q1_13 : Outport  Port=19  VectorParamsAs1DForOutWhenUnconnected=off
  Q1_21 : Outport  Port=20  VectorParamsAs1DForOutWhenUnconnected=off
  Q1_22 : Outport  Port=21  VectorParamsAs1DForOutWhenUnconnected=off
  C_1 : Outport  Port=22  VectorParamsAs1DForOutWhenUnconnected=off
  C_2 : Outport  Port=23  VectorParamsAs1DForOutWhenUnconnected=off
  wires:
  Mux/1 -> Mux1/1
  Mux1/1 -> Modbus Write/1
  Constant/1 -> Mux1/2
  Demux1/5 -> P_22/1
  V_12/1 -> Mux/2
  Demux1/6 -> P_23/1
  Demux1/3 -> P_13/1
  Demux1/4 -> P_21/1
  V_13/1 -> Mux/3
  Demux3/2 -> Q1_12/1
  Demux3/5 -> Q1_22/1
  Demux/2 -> dP_2/1
  Demux3/1 -> Q1_11/1
  Demux1/2 -> P_12/1
  Demux2/5 -> T_25/1
  Demux4/1 -> C_1/1
  V_21/1 -> Mux/4
  Demux3/3 -> Q1_13/1
  Demux1/1 -> P_11/1
  Demux3/4 -> Q1_21/1
  V_11/1 -> Mux/1
  Demux2/4 -> T_24/1
  Demux2/3 -> T_23/1
  Demux2/2 -> T_22/1
  Demux2/1 -> T_21/1
  Demux1/7 -> P_24/1
  V_22/1 -> Mux/5
  Demux2/7 -> T_27/1
  Demux/5 -> Demux4/1
  Demux/1 -> Demux1/1
  Demux2/8 -> T_28/1
  Demux4/2 -> C_2/1
  Demux/3 -> Demux2/1
  Demux/4 -> Demux3/1
  Modbus Read/1 -> Demux/1
  Demux2/6 -> T_26/1

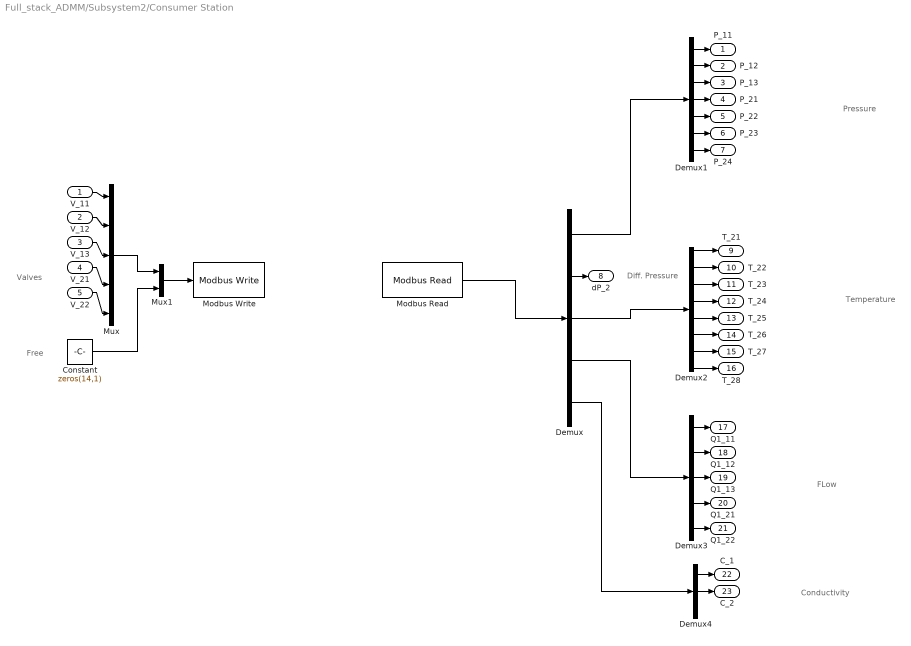
== system Full_stack_ADMM/Subsystem2/Consumer Station ==
  note: Free
  note: Diff. Pressure
  note: Valves
  note: Conductivity
  note: FLow
  note: Temperature
  note: Pressure
  V_11 : Inport
  V_12 : Inport  Port=2
  V_13 : Inport  Port=3
  V_21 : Inport  Port=4
  V_22 : Inport  Port=5
  Constant : Constant  Value=zeros(14,1)
  Demux : Demux  Outputs=[7 1 8 5 3]
  Demux1 : Demux  Outputs=7
  Demux2 : Demux  Outputs=8
  Demux3 : Demux  Outputs=5
  Demux4 : Demux  Outputs=3
  Modbus Read : modbusMatLib/Modbus Read  registry=0  ipAddress='192.168.100.32'  port=502
  Modbus Write : modbusMatLib/Modbus Write  registry=001  port=502  ipAddress='192.168.100.32'
  Mux : Mux  Inputs=5
  Mux1 : Mux  Inputs=2
  P_11 : Outport  VectorParamsAs1DForOutWhenUnconnected=off
  P_12 : Outport  Port=2  VectorParamsAs1DForOutWhenUnconnected=off
  P_13 : Outport  Port=3  VectorParamsAs1DForOutWhenUnconnected=off
  P_21 : Outport  Port=4  VectorParamsAs1DForOutWhenUnconnected=off
  P_22 : Outport  Port=5  VectorParamsAs1DForOutWhenUnconnected=off
  P_23 : Outport  Port=6  VectorParamsAs1DForOutWhenUnconnected=off
  P_24 : Outport  Port=7  VectorParamsAs1DForOutWhenUnconnected=off
  dP_2 : Outport  Port=8  VectorParamsAs1DForOutWhenUnconnected=off
  T_21 : Outport  Port=9  VectorParamsAs1DForOutWhenUnconnected=off
  T_22 : Outport  Port=10  VectorParamsAs1DForOutWhenUnconnected=off
  T_23 : Outport  Port=11  VectorParamsAs1DForOutWhenUnconnected=off
  T_24 : Outport  Port=12  VectorParamsAs1DForOutWhenUnconnected=off
  T_25 : Outport  Port=13  VectorParamsAs1DForOutWhenUnconnected=off
  T_26 : Outport  Port=14  VectorParamsAs1DForOutWhenUnconnected=off
  T_27 : Outport  Port=15  VectorParamsAs1DForOutWhenUnconnected=off
  T_28 : Outport  Port=16  VectorParamsAs1DForOutWhenUnconnected=off
  Q1_11 : Outport  Port=17  VectorParamsAs1DForOutWhenUnconnected=off
  Q1_12 : Outport  Port=18  VectorParamsAs1DForOutWhenUnconnected=off
  Q1_13 : Outport  Port=19  VectorParamsAs1DForOutWhenUnconnected=off
  Q1_21 : Outport  Port=20  VectorParamsAs1DForOutWhenUnconnected=off
  Q1_22 : Outport  Port=21  VectorParamsAs1DForOutWhenUnconnected=off
  C_1 : Outport  Port=22  VectorParamsAs1DForOutWhenUnconnected=off
  C_2 : Outport  Port=23  VectorParamsAs1DForOutWhenUnconnected=off
  wires:
  Demux2/6 -> T_26/1
  Modbus Read/1 -> Demux/1
  Demux/4 -> Demux3/1
  Demux/3 -> Demux2/1
  Demux4/2 -> C_2/1
  Demux2/8 -> T_28/1
  Demux/1 -> Demux1/1
  Demux/5 -> Demux4/1
  Demux2/7 -> T_27/1
  V_22/1 -> Mux/5
  Demux1/7 -> P_24/1
  Demux2/1 -> T_21/1
  Demux2/2 -> T_22/1
  Demux2/3 -> T_23/1
  Demux2/4 -> T_24/1
  V_11/1 -> Mux/1
  Demux3/4 -> Q1_21/1
  Demux1/1 -> P_11/1
  Demux3/3 -> Q1_13/1
  V_21/1 -> Mux/4
  Demux4/1 -> C_1/1
  Demux2/5 -> T_25/1
  Demux1/2 -> P_12/1
  Demux3/1 -> Q1_11/1
  Demux/2 -> dP_2/1
  Demux3/5 -> Q1_22/1
  Demux3/2 -> Q1_12/1
  V_13/1 -> Mux/3
  Demux1/4 -> P_21/1
  Demux1/3 -> P_13/1
  Demux1/6 -> P_23/1
  V_12/1 -> Mux/2
  Demux1/5 -> P_22/1
  Constant/1 -> Mux1/2
  Mux1/1 -> Modbus Write/1
  Mux/1 -> Mux1/1

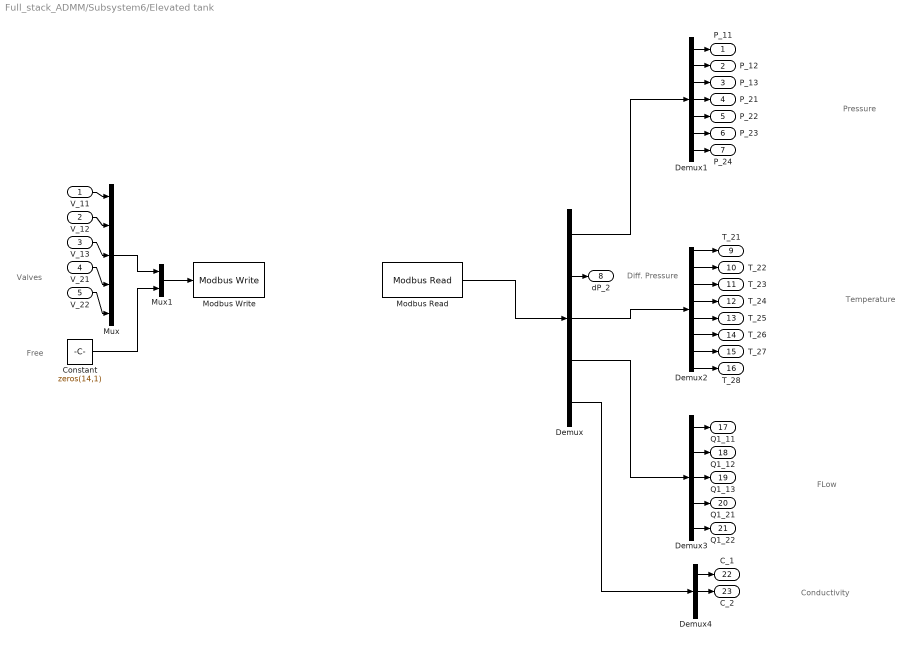
== system Full_stack_ADMM/Subsystem6/Elevated tank ==
  note: Pressure
  note: Temperature
  note: FLow
  note: Conductivity
  note: Valves
  note: Diff. Pressure
  note: Free
  V_11 : Inport
  V_12 : Inport  Port=2
  V_13 : Inport  Port=3
  V_21 : Inport  Port=4
  V_22 : Inport  Port=5
  Constant : Constant  Value=zeros(14,1)
  Demux : Demux  Outputs=[7 1 8 5 3]
  Demux1 : Demux  Outputs=7
  Demux2 : Demux  Outputs=8
  Demux3 : Demux  Outputs=5
  Demux4 : Demux  Outputs=3
  Modbus Read : modbusMatLib/Modbus Read  registry=0  ipAddress='192.168.100.34'  port=502
  Modbus Write : modbusMatLib/Modbus Write  registry=001  port=502  ipAddress='192.168.100.34'
  Mux : Mux  Inputs=5
  Mux1 : Mux  Inputs=2
  P_11 : Outport  VectorParamsAs1DForOutWhenUnconnected=off
  P_12 : Outport  Port=2  VectorParamsAs1DForOutWhenUnconnected=off
  P_13 : Outport  Port=3  VectorParamsAs1DForOutWhenUnconnected=off
  P_21 : Outport  Port=4  VectorParamsAs1DForOutWhenUnconnected=off
  P_22 : Outport  Port=5  VectorParamsAs1DForOutWhenUnconnected=off
  P_23 : Outport  Port=6  VectorParamsAs1DForOutWhenUnconnected=off
  P_24 : Outport  Port=7  VectorParamsAs1DForOutWhenUnconnected=off
  dP_2 : Outport  Port=8  VectorParamsAs1DForOutWhenUnconnected=off
  T_21 : Outport  Port=9  VectorParamsAs1DForOutWhenUnconnected=off
  T_22 : Outport  Port=10  VectorParamsAs1DForOutWhenUnconnected=off
  T_23 : Outport  Port=11  VectorParamsAs1DForOutWhenUnconnected=off
  T_24 : Outport  Port=12  VectorParamsAs1DForOutWhenUnconnected=off
  T_25 : Outport  Port=13  VectorParamsAs1DForOutWhenUnconnected=off
  T_26 : Outport  Port=14  VectorParamsAs1DForOutWhenUnconnected=off
  T_27 : Outport  Port=15  VectorParamsAs1DForOutWhenUnconnected=off
  T_28 : Outport  Port=16  VectorParamsAs1DForOutWhenUnconnected=off
  Q1_11 : Outport  Port=17  VectorParamsAs1DForOutWhenUnconnected=off
  Q1_12 : Outport  Port=18  VectorParamsAs1DForOutWhenUnconnected=off
  Q1_13 : Outport  Port=19  VectorParamsAs1DForOutWhenUnconnected=off
  Q1_21 : Outport  Port=20  VectorParamsAs1DForOutWhenUnconnected=off
  Q1_22 : Outport  Port=21  VectorParamsAs1DForOutWhenUnconnected=off
  C_1 : Outport  Port=22  VectorParamsAs1DForOutWhenUnconnected=off
  C_2 : Outport  Port=23  VectorParamsAs1DForOutWhenUnconnected=off
  wires:
  Mux/1 -> Mux1/1
  Mux1/1 -> Modbus Write/1
  Constant/1 -> Mux1/2
  Demux1/5 -> P_22/1
  V_12/1 -> Mux/2
  Demux1/6 -> P_23/1
  Demux1/3 -> P_13/1
  Demux1/4 -> P_21/1
  V_13/1 -> Mux/3
  Demux3/2 -> Q1_12/1
  Demux3/5 -> Q1_22/1
  Demux/2 -> dP_2/1
  Demux3/1 -> Q1_11/1
  Demux1/2 -> P_12/1
  Demux2/5 -> T_25/1
  Demux4/1 -> C_1/1
  V_21/1 -> Mux/4
  Demux3/3 -> Q1_13/1
  Demux1/1 -> P_11/1
  Demux3/4 -> Q1_21/1
  V_11/1 -> Mux/1
  Demux2/4 -> T_24/1
  Demux2/3 -> T_23/1
  Demux2/2 -> T_22/1
  Demux2/1 -> T_21/1
  Demux1/7 -> P_24/1
  V_22/1 -> Mux/5
  Demux2/7 -> T_27/1
  Demux/5 -> Demux4/1
  Demux/1 -> Demux1/1
  Demux2/8 -> T_28/1
  Demux4/2 -> C_2/1
  Demux/3 -> Demux2/1
  Demux/4 -> Demux3/1
  Modbus Read/1 -> Demux/1
  Demux2/6 -> T_26/1
